simulink model "online_ups_simulation"  (R2025b)
settings: Solver=ode4  StartTime=0.0  StopTime=1  FixedStep=1e-6  MaxStep=1e-5  RelTol=1e-3
undefined symbols (not defined in the file): Ion, Lithium
libraries: spsSeriesRLCBranchLib x6, spsACVoltageSourceLib x2, spsIdealSwitchLib x2, spsUniversalBridgeLib x2, spsBatteryLib x1, spsCurrentMeasurementLib x1, simulink x1, spsSeriesRLCLoadLib x1, spsTwoQuadrantDCDCConverterLib x1, spsVoltageMeasurementLib x1, sps_lib x1
settings Model: Creator=ADMIN  LastModifiedBy=ADMIN

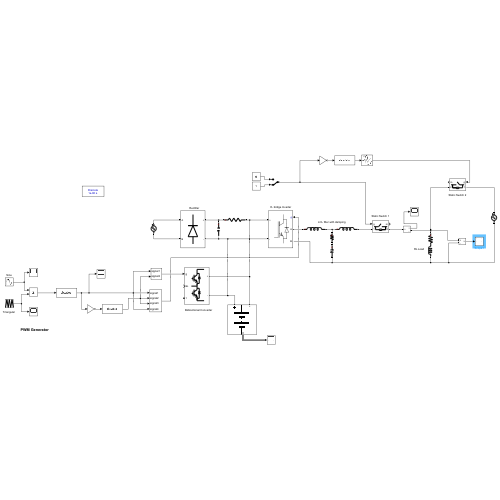
[thumbnail: Simulink's stored preview of the top-level diagram]
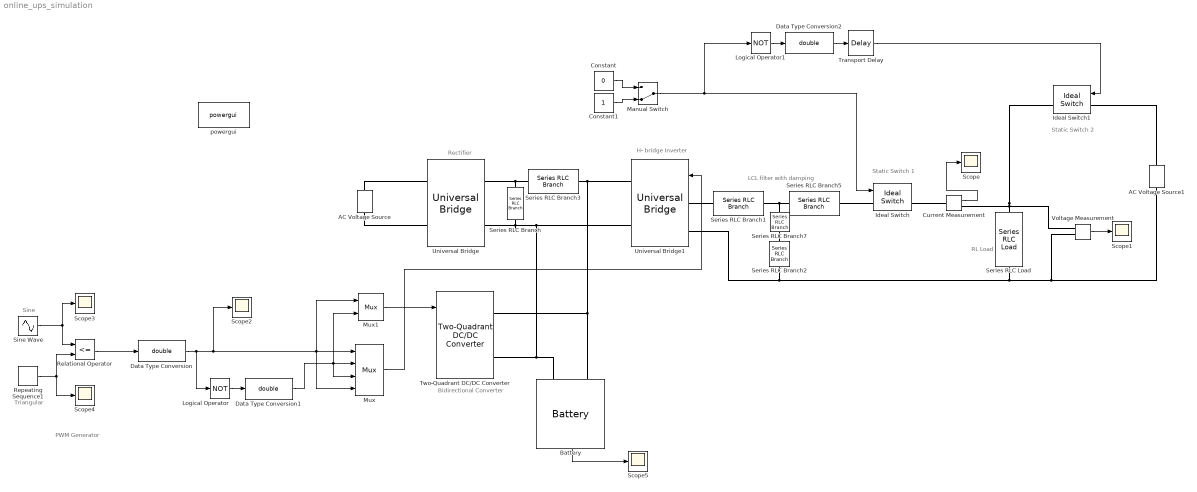
== system online_ups_simulation ==
  note: Static Switch 1
  note: Bidirectional Converter
  note: PWM Generator
  note: LCL filter with damping
  note: Triangular
  note: Sine
  note: RL Load
  note: Rectifier
  note: H- bridge Inverter
  note: Static Switch 2
  AC Voltage Source : spsACVoltageSourceLib/AC Voltage Source  Amplitude=325  Phase=0  Frequency=50  SampleTime=0  Measurements=None  BusType=swing  Pref=10e3  Qref=0  Qmin=-inf  Qmax=+inf
  AC Voltage Source1 : spsACVoltageSourceLib/AC Voltage Source  Amplitude=325  Phase=0  Frequency=50  SampleTime=0  Measurements=None  BusType=swing  Pref=10e3  Qref=0  Qmin=-inf  Qmax=+inf
  Battery : spsBatteryLib/Battery  BatType=Lithium-Ion  NomV=360  NomQ=5.4  SOC=100  Batt_Tr=30  PresetModel=on  MaxQ=5.4  MinV=270  FullV=419.0354  Dis_rate=2.3478  R=0.66667  Normal_OP=4.8835  expZone="[388.9389     0.2653043]"
  Constant : Constant  Value=0
  Constant1 : Constant
  Current Measurement : spsCurrentMeasurementLib/Current Measurement  PhasorSimulation=off  OutputType=Complex  PSBequivalent=0
  Data Type Conversion : DataTypeConversion  OutMin=0  OutMax=1  OutDataTypeStr=double  SaturateOnIntegerOverflow=off  RndMeth=Floor
  Data Type Conversion1 : DataTypeConversion  OutMin=0  OutMax=1  OutDataTypeStr=double  SaturateOnIntegerOverflow=off  RndMeth=Floor
  Data Type Conversion2 : DataTypeConversion  OutMin=0  OutMax=1  OutDataTypeStr=double  SaturateOnIntegerOverflow=off  RndMeth=Floor
  Ideal Switch : spsIdealSwitchLib/Ideal Switch  Ron=0.01  Lon=0  IC=0  Rs=1e5  Cs=inf  Measurements=on
  Ideal Switch1 : spsIdealSwitchLib/Ideal Switch  Ron=0.01  Lon=0  IC=0  Rs=1e5  Cs=inf  Measurements=on
  Logical Operator : Logic  Operator=NOT  IconShape=distinctive  AllPortsSameDT=off  OutDataTypeStr=boolean
  Logical Operator1 : Logic  Operator=NOT  IconShape=distinctive  AllPortsSameDT=off  OutDataTypeStr=boolean
  Manual Switch : ManualSwitch  CurrentSetting=0
  Mux : Mux
      settings: DisplayOption=signals
  Mux1 : Mux  Inputs=2
      settings: DisplayOption=signals
  Relational Operator : RelationalOperator  Operator=<=  OutDataTypeStr=boolean  RndMeth=Simplest  InputSameDT=off
  Repeating Sequence1 : simulink/Sources/Repeating Sequence  rep_seq_t=[0 0.0001 0.0002]  rep_seq_y=[-1 1 -1]
  Scope{,1..5} (6 alike) : Scope
      Scope settings: ActiveDisplayYMinimum=-4.8010833627671907  ActiveDisplayYMaximum=5.4091370970408654
      Scope1 settings: ActiveDisplayYMinimum=-586.75892943278882  ActiveDisplayYMaximum=502.85352835914233
      Scope2 settings: ActiveDisplayYMinimum=0.4346411559950506  ActiveDisplayYMaximum=0.51758651536372258  DataLoggingVariableName=ScopeData2
      Scope3 settings: ActiveDisplayYMinimum=-9.78668131778553  ActiveDisplayYMaximum=8.3539082513754757  DataLoggingVariableName=ScopeData3
      Scope4 settings: ActiveDisplayYMinimum=-1.0611299389064666  ActiveDisplayYMaximum=1.2760967483323333  DataLoggingVariableName=ScopeData4
      Scope5 settings: ActiveDisplayYMinimum=-565.77077697515313  ActiveDisplayYMaximum=1364.594209190388  DataLoggingVariableName=ScopeData5
  Series RLC Branch : spsSeriesRLCBranchLib/Series RLC Branch  LConnTagsString=__new0  RConnTagsString=__new0  BranchType=C  Resistance=1  Inductance=1e-3  SetiL0=off  InitialCurrent=0  Capacitance=2.2e-3  Setx0=off  InitialVoltage=0  Measurements=None
  Series RLC Branch1 : spsSeriesRLCBranchLib/Series RLC Branch  LConnTagsString=__new0  RConnTagsString=__new0  BranchType=L  Resistance=0  Inductance=3e-3  SetiL0=off  InitialCurrent=0  Capacitance=0  Setx0=off  InitialVoltage=0  Measurements=None
  Series RLC Branch2 : spsSeriesRLCBranchLib/Series RLC Branch  LConnTagsString=__new0  RConnTagsString=__new0  BranchType=C  Resistance=0  Inductance=0  SetiL0=off  InitialCurrent=0  Capacitance=10e-6  Setx0=off  InitialVoltage=0  Measurements=None
  Series RLC Branch3 : spsSeriesRLCBranchLib/Series RLC Branch  LConnTagsString=__new0  RConnTagsString=__new0  BranchType=R  Resistance=0.05  Inductance=3e-3  SetiL0=off  InitialCurrent=0  Capacitance=0  Setx0=off  InitialVoltage=0  Measurements=None
  Series RLC Branch5 : spsSeriesRLCBranchLib/Series RLC Branch  LConnTagsString=__new0  RConnTagsString=__new0  BranchType=L  Resistance=0  Inductance=3e-3  SetiL0=off  InitialCurrent=0  Capacitance=0  Setx0=off  InitialVoltage=0  Measurements=None
  Series RLC Branch7 : spsSeriesRLCBranchLib/Series RLC Branch  LConnTagsString=__new0  RConnTagsString=__new0  BranchType=R  Resistance=5  Inductance=5e-3  SetiL0=off  InitialCurrent=0  Capacitance=0  Setx0=off  InitialVoltage=0  Measurements=None
  Series RLC Load : spsSeriesRLCLoadLib/Series RLC Load  LConnTagsString=a  RConnTagsString=__new0  NominalVoltage=230  NominalFrequency=50  ActivePower=500  InductivePower=100  CapacitivePower=0  Setx0=off  InitialVoltage=0  SetiL0=off  InitialCurrent=0  Measurements=None  LoadType=constant Z
  Sine Wave : Sin  Amplitude=0.8  Frequency=2*pi*50  SampleTime=1e-5
  Transport Delay : TransportDelay  DelayTime=1e-3
  Two-Quadrant DC/DC Converter : spsTwoQuadrantDCDCConverterLib/Two-Quadrant DC//DC Converter  ModelType=Switching devices  Ron=1e-3  Rs=1e6  Cs=inf  Vforward=[0,0]  Ron_Diode=1e-3  Rs_Diode=1e6  Cs_Diode=inf  Vf_Diode=1e-3  Rs_CurrentSource=inf  Ron_ACsource=1e-3
  Universal Bridge : spsUniversalBridgeLib/Universal Bridge  Arms=2  SnubberResistance=1e5  SnubberCapacitance=inf  Device=Diodes  Ron=1e-3  Lon=0  ForwardVoltages="[  0  0  ]"  ForwardVoltage=0  GTOparameters=[ 10e-6 , 20e-6 ]  IGBTparameters=[ 1e-6 , 2e-6 ]  Measurements=None  Measurements_2=None  converterType=Rectifier
  Universal Bridge1 : spsUniversalBridgeLib/Universal Bridge  Arms=2  SnubberResistance=1e5  SnubberCapacitance=inf  Device=IGBT / Diodes  Ron=1e-3  Lon=0  ForwardVoltages="[  0  0  ]"  ForwardVoltage=0  GTOparameters=[ 10e-6 , 20e-6 ]  IGBTparameters=[ 1e-6 , 2e-6 ]  Measurements=None  Measurements_2=None  converterType=Rectifier
  Voltage Measurement : spsVoltageMeasurementLib/Voltage Measurement  PhasorSimulation=off  OutputType=Complex  PSBequivalent=0
  powergui : sps_lib/powergui  Priority=1  SimulationMode=Discrete  SampleTime=1e-6  frequency=60  Iterations=50  frequencyindice=50  Pbase=100e6  ErrMax=1e-4  UnitsV=kV  UnitsW=MW  buscounter=0  FunctionMessages=off  echomessages=off  EnableUseOfTLC=off  CurrentSourceSwitches=off  DisableSnubberDevices=off  DisableRonSwitches=off  DisableVfSwitches=off  DisplayEquations=off  AutomaticDiscreteSolvers=off  SolverType=Tustin/Backward Euler (TBE)  Interpol=off  ExternalGateDelay=off  methode=off  Ts=100  x0status=blocks  SPID=on  SwTol=0  HookPort=off  NonlinearTolerance=1e-4  nMaxIteration=100  ContinueOnMaxIteration=off  RestoreLinks=warning  ResistiveCurrentMeasurement=off  Frange=[0:2:500]  Ylog=off  Xlog=on  ShowGrid=off  save=off  variable=ZData  structure=0  ZoomFFT=off  StartTime=0.0  cycles=1  DisplayStyle=1  fundamental=60  FreqAxis=off  MaxFrequency=1000  frequencyindicesteady=1  RmsSteady=1  display=off
  wires:
  Sine Wave/1 -> Scope3/1, Relational Operator/1
  Voltage Measurement/1 -> Scope1/1
  Current Measurement/1 -> Scope/1
  Mux/1 -> Universal Bridge1/1
  Relational Operator/1 -> Data Type Conversion/1
  Data Type Conversion/1 -> Scope2/1, Mux1/1, Mux/4, Mux/1, Logical Operator/1
  Logical Operator/1 -> Data Type Conversion1/1
  Repeating Sequence1/1 -> Scope4/1, Relational Operator/2
  Data Type Conversion1/1 -> Mux/3, Mux/2, Mux1/2
  Mux1/1 -> Two-Quadrant DC/DC Converter/1
  Constant/1 -> Manual Switch/1
  Constant1/1 -> Manual Switch/2
  Transport Delay/1 -> Ideal Switch1/1
  Battery/1 -> Scope5/1
  Manual Switch/1 -> Logical Operator1/1, Ideal Switch/1
  Logical Operator1/1 -> Data Type Conversion2/1
  Data Type Conversion2/1 -> Transport Delay/1
  connections:
  AC Voltage Source/RConn1 -- Universal Bridge/LConn1
  AC Voltage Source/LConn1 -- Universal Bridge/LConn2
  Battery/LConn1 -- Universal Bridge1/RConn1 -- Series RLC Branch3/RConn1 -- Two-Quadrant DC/DC Converter/RConn1
  Series RLC Branch1/LConn1 -- Universal Bridge1/LConn1
  Series RLC Branch7/LConn1 -- Series RLC Branch1/RConn1 -- Series RLC Branch5/LConn1
  Series RLC Branch2/RConn1 -- Universal Bridge1/LConn2 -- AC Voltage Source1/LConn1 -- Voltage Measurement/LConn2 -- Series RLC Load/RConn1
  Universal Bridge/RConn2 -- Series RLC Branch/RConn1 -- Two-Quadrant DC/DC Converter/RConn2 -- Battery/LConn2 -- Universal Bridge1/RConn2
  Series RLC Branch7/RConn1 -- Series RLC Branch2/LConn1
  Universal Bridge/RConn1 -- Series RLC Branch3/LConn1 -- Series RLC Branch/LConn1
  Series RLC Branch5/RConn1 -- Ideal Switch/LConn1
  Current Measurement/RConn1 -- Ideal Switch1/RConn1 -- Series RLC Load/LConn1 -- Voltage Measurement/LConn1
  Ideal Switch/RConn1 -- Current Measurement/LConn1
  Ideal Switch1/LConn1 -- AC Voltage Source1/RConn1
